simulink model "saccha"  (Simulink 6.4)
settings: Solver=ode15s  StartTime=0.0  StopTime=35  FixedStep=1  RelTol=1e-3
values from neighbouring files (symbols this model uses):
  med_err = 5    [saccha.mat]    (also in simule.m)
  r = [66 49 41 5 78 55 23 52 31 162]    [saccha.mat]    (also in simule.m = round(abs(100*randn(10,1))))
settings Model: LastModifiedBy=jcamacho
settings DataIOCC: LimitDataPoints=off  SignalLoggingName=sigsOut
settings DebuggingCC: SolverPrmCheckMsg=none  StrictBusMsg=None
settings HardwareCC: TargetUnknown=on

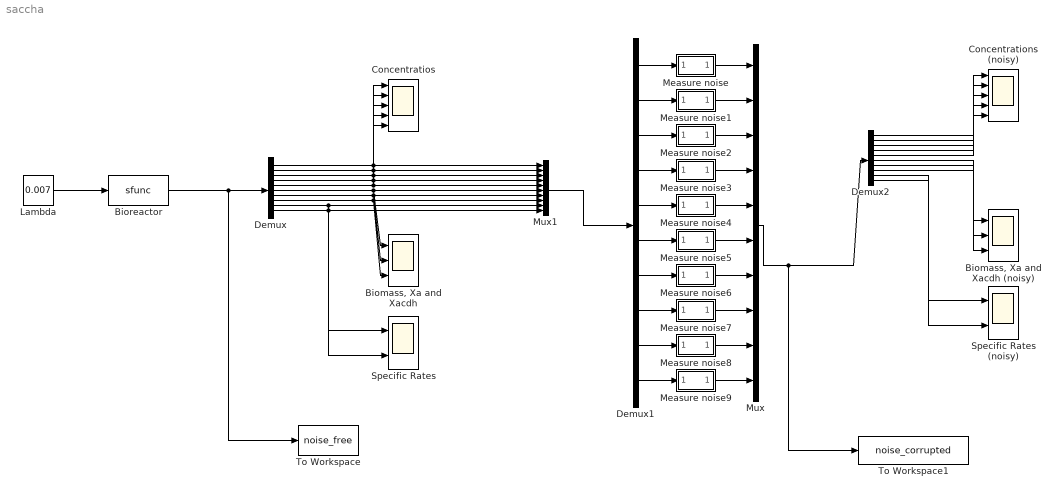
== system saccha ==
  "Biomass, Xa and Xacdh " : Scope  NumInputPorts=3
      settings: TimeRange=10  YMin=28.8275~0.9~1  YMax=28.86~1~1.04  MaxDataPoints=100000
  "Biomass, Xa and Xacdh (noisy)" : Scope  NumInputPorts=3
      settings: TimeRange=10  YMin=0.6~0.9~1  YMax=1~1~1.04  SaveName=ScopeData3  MaxDataPoints=40000
  Bioreactor : S-Function  FunctionName=sfunc  Parameters=xini, k1h, K1h, k1l, K1l, k1e, K1e, K1i, k2, K2, K2i, k3, K3, k4, K4, k5, K5, k5e, K5e, K5i, k6, K6, k6r, K6e, k7, K7, k8, k9, K9, k9e, K9e, K9i, k9c, k10, K10, k10e, K10e, k11, Sf, w, var_ini
  Concentrations (noisy) : Scope  NumInputPorts=5
      settings: TimeRange=10  YMin=0.6~0.9~1~1~0  YMax=1~1~1.04~1.001~100  SaveName=ScopeData5  MaxDataPoints=40000
  Concentratios : Scope  NumInputPorts=5
      settings: TimeRange=1  YMin=0.6~0.9~1~1~0  YMax=1~1~1.04~1.001~100  MaxDataPoints=40000
  Demux : Demux  Outputs=10
  Demux1 : Demux  Outputs=10
  Demux2 : Demux  Outputs=10
  Lambda : Constant  Value=0.007  OutDataType=sfix(16)  ConRadixGroup=Use specified scaling  OutScaling=2^0  SampleTime=inf  FramePeriod=inf
  Measure noise : Subsystem  TreatAsAtomicUnit=on  mask{v1=0, v2=15*med_err/200, v3=0, v4=r(1)}
      mask prompts: v1 "Media error blanco"; v2 "Desviacion Tipica error blanco"; v3 "Constante de error proporcional"; v4 "Semilla"
      mask init:
      | media = v1;
      | varianza = v2*v2;
      | proporcional = v3;
      | r = v4;
  Measure noise1 : Subsystem  TreatAsAtomicUnit=on  mask{v1=0, v2=0.02*med_err/200, v3=0, v4=r(2)}
      mask prompts: v1 "Media error blanco"; v2 "Desviacion Tipica error blanco"; v3 "Constante de error proporcional"; v4 "Semilla"
      mask init:
      | media = v1;
      | varianza = v2*v2;
      | proporcional = v3;
      | r = v4;
  Measure noise2 : Subsystem  TreatAsAtomicUnit=on  mask{v1=0, v2=1*med_err/200, v3=0, v4=r(3)}
      mask prompts: v1 "Media error blanco"; v2 "Desviacion Tipica error blanco"; v3 "Constante de error proporcional"; v4 "Semilla"
      mask init:
      | media = v1;
      | varianza = v2*v2;
      | proporcional = v3;
      | r = v4;
  Measure noise3 : Subsystem  TreatAsAtomicUnit=on  mask{v1=0, v2=0.05*med_err/200, v3=0, v4=r(4)}
      mask prompts: v1 "Media error blanco"; v2 "Desviacion Tipica error blanco"; v3 "Constante de error proporcional"; v4 "Semilla"
      mask init:
      | media = v1;
      | varianza = v2*v2;
      | proporcional = v3;
      | r = v4;
  Measure noise4 : Subsystem  TreatAsAtomicUnit=on  mask{v1=0, v2=5*med_err/200, v3=0, v4=r(5)}
      mask prompts: v1 "Media error blanco"; v2 "Desviacion Tipica error blanco"; v3 "Constante de error proporcional"; v4 "Semilla"
      mask init:
      | media = v1;
      | varianza = v2*v2;
      | proporcional = v3;
      | r = v4;
  Measure noise5 : Subsystem  TreatAsAtomicUnit=on  mask{v1=0, v2=2.5*med_err/200, v3=0, v4=r(6)}
      mask prompts: v1 "Media error blanco"; v2 "Desviacion Tipica error blanco"; v3 "Constante de error proporcional"; v4 "Semilla"
      mask init:
      | media = v1;
      | varianza = v2*v2;
      | proporcional = v3;
      | r = v4;
  Measure noise6 : Subsystem  TreatAsAtomicUnit=on  mask{v1=0, v2=0.1*med_err/200, v3=0, v4=r(7)}
      mask prompts: v1 "Media error blanco"; v2 "Desviacion Tipica error blanco"; v3 "Constante de error proporcional"; v4 "Semilla"
      mask init:
      | media = v1;
      | varianza = v2*v2;
      | proporcional = v3;
      | r = v4;
  Measure noise7 : Subsystem  TreatAsAtomicUnit=on  mask{v1=0, v2=0.02*med_err/200, v3=0, v4=r(8)}
      mask prompts: v1 "Media error blanco"; v2 "Desviacion Tipica error blanco"; v3 "Constante de error proporcional"; v4 "Semilla"
      mask init:
      | media = v1;
      | varianza = v2*v2;
      | proporcional = v3;
      | r = v4;
  Measure noise8 : Subsystem  TreatAsAtomicUnit=on  mask{v1=0, v2=5*med_err/200, v3=0, v4=r(9)}
      mask prompts: v1 "Media error blanco"; v2 "Desviacion Tipica error blanco"; v3 "Constante de error proporcional"; v4 "Semilla"
      mask init:
      | media = v1;
      | varianza = v2*v2;
      | proporcional = v3;
      | r = v4;
  Measure noise9 : Subsystem  TreatAsAtomicUnit=on  mask{v1=0, v2=15*med_err/200, v3=0, v4=r(10)}
      mask prompts: v1 "Media error blanco"; v2 "Desviacion Tipica error blanco"; v3 "Constante de error proporcional"; v4 "Semilla"
      mask init:
      | media = v1;
      | varianza = v2*v2;
      | proporcional = v3;
      | r = v4;
  Mux : Mux  Inputs=10
  Mux1 : Mux  Inputs=10
  Specific Rates : Scope  NumInputPorts=2
      settings: TimeRange=10  YMin=0.6~1.38778e-017  YMax=1~0.375  SaveName=ScopeData2  MaxDataPoints=40000
  Specific Rates (noisy) : Scope  NumInputPorts=2
      settings: TimeRange=10  YMin=0.6~0.9  YMax=1~1  SaveName=ScopeData4  MaxDataPoints=40000
  To Workspace : ToWorkspace  VariableName=noise_free  SampleTime=-1  SaveFormat=Structure With Time
  To Workspace1 : ToWorkspace  VariableName=noise_corrupted  SampleTime=-1  SaveFormat=Structure With Time
  wires:
  Demux/1 -> Concentratios/1, Mux1/1
  Demux/2 -> Concentratios/2, Mux1/2
  Demux/3 -> Concentratios/3, Mux1/3
  Demux/4 -> Concentratios/4, Mux1/4
  Demux/5 -> Concentratios/5, Mux1/5
  Demux/6 -> "Biomass, Xa and Xacdh "/1, Mux1/6
  Demux/7 -> "Biomass, Xa and Xacdh "/2, Mux1/7
  Demux/8 -> "Biomass, Xa and Xacdh "/3, Mux1/8
  Bioreactor/1 -> Demux/1, To Workspace/1
  Demux1/1 -> Measure noise/1(In1)
  Demux1/2 -> Measure noise1/1(In1)
  Demux1/3 -> Measure noise2/1(In1)
  Demux1/4 -> Measure noise3/1(In1)
  Demux1/5 -> Measure noise4/1(In1)
  Demux1/6 -> Measure noise5/1(In1)
  Demux1/7 -> Measure noise6/1(In1)
  Demux1/8 -> Measure noise7/1(In1)
  Measure noise/1(Out1) -> Mux/1
  Measure noise1/1(Out1) -> Mux/2
  Measure noise2/1(Out1) -> Mux/3
  Measure noise3/1(Out1) -> Mux/4
  Measure noise4/1(Out1) -> Mux/5
  Measure noise5/1(Out1) -> Mux/6
  Measure noise6/1(Out1) -> Mux/7
  Measure noise7/1(Out1) -> Mux/8
  Measure noise8/1(Out1) -> Mux/9
  Measure noise9/1(Out1) -> Mux/10
  Demux2/1 -> Concentrations (noisy)/1
  Demux2/2 -> Concentrations (noisy)/2
  Demux2/3 -> Concentrations (noisy)/3
  Demux2/4 -> Concentrations (noisy)/4
  Demux2/5 -> Concentrations (noisy)/5
  Demux2/6 -> "Biomass, Xa and Xacdh (noisy)"/1
  Demux2/7 -> "Biomass, Xa and Xacdh (noisy)"/2
  Demux2/8 -> "Biomass, Xa and Xacdh (noisy)"/3
  Demux2/9 -> Specific Rates (noisy)/1
  Demux2/10 -> Specific Rates (noisy)/2
  Mux/1 -> Demux2/1, To Workspace1/1
  Demux1/9 -> Measure noise8/1(In1)
  Demux1/10 -> Measure noise9/1(In1)
  Demux/9 -> Specific Rates/1, Mux1/9
  Demux/10 -> Specific Rates/2, Mux1/10
  Mux1/1 -> Demux1/1
  Lambda/1 -> Bioreactor/1

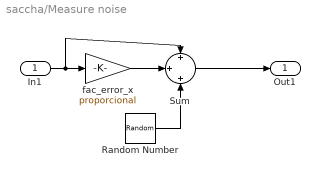
== system saccha/Measure noise ==
  In1 : Inport
  Random Number : RandomNumber  Mean=media  Variance=varianza  Seed=r  SampleTime=0
  Sum : Sum  Inputs=+|+|+  SaturateOnIntegerOverflow=on
  fac_error_x : Gain  Gain=proporcional  SaturateOnIntegerOverflow=on
  Out1 : Outport
  wires:
  Random Number/1 -> Sum/3
  In1/1 -> fac_error_x/1, Sum/1
  fac_error_x/1 -> Sum/2
  Sum/1 -> Out1/1

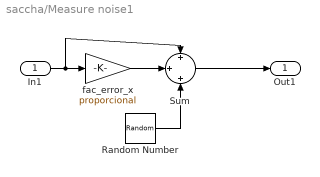
== system saccha/Measure noise1 ==
  In1 : Inport
  Random Number : RandomNumber  Mean=media  Variance=varianza  Seed=r  SampleTime=0
  Sum : Sum  Inputs=+|+|+  SaturateOnIntegerOverflow=on
  fac_error_x : Gain  Gain=proporcional  SaturateOnIntegerOverflow=on
  Out1 : Outport
  wires:
  Random Number/1 -> Sum/3
  In1/1 -> fac_error_x/1, Sum/1
  fac_error_x/1 -> Sum/2
  Sum/1 -> Out1/1

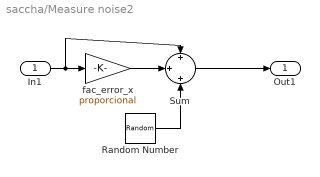
== system saccha/Measure noise2 ==
  In1 : Inport
  Random Number : RandomNumber  Mean=media  Variance=varianza  Seed=r  SampleTime=0
  Sum : Sum  Inputs=+|+|+  SaturateOnIntegerOverflow=on
  fac_error_x : Gain  Gain=proporcional  SaturateOnIntegerOverflow=on
  Out1 : Outport
  wires:
  Random Number/1 -> Sum/3
  In1/1 -> fac_error_x/1, Sum/1
  fac_error_x/1 -> Sum/2
  Sum/1 -> Out1/1

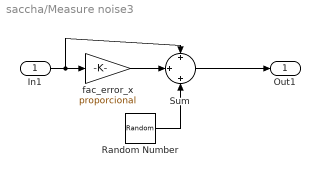
== system saccha/Measure noise3 ==
  In1 : Inport
  Random Number : RandomNumber  Mean=media  Variance=varianza  Seed=r  SampleTime=0
  Sum : Sum  Inputs=+|+|+  SaturateOnIntegerOverflow=on
  fac_error_x : Gain  Gain=proporcional  SaturateOnIntegerOverflow=on
  Out1 : Outport
  wires:
  Random Number/1 -> Sum/3
  In1/1 -> fac_error_x/1, Sum/1
  fac_error_x/1 -> Sum/2
  Sum/1 -> Out1/1

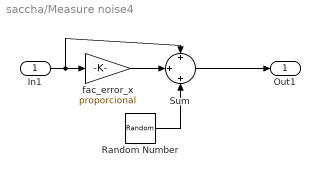
== system saccha/Measure noise4 ==
  In1 : Inport
  Random Number : RandomNumber  Mean=media  Variance=varianza  Seed=r  SampleTime=0
  Sum : Sum  Inputs=+|+|+  SaturateOnIntegerOverflow=on
  fac_error_x : Gain  Gain=proporcional  SaturateOnIntegerOverflow=on
  Out1 : Outport
  wires:
  Random Number/1 -> Sum/3
  In1/1 -> fac_error_x/1, Sum/1
  fac_error_x/1 -> Sum/2
  Sum/1 -> Out1/1

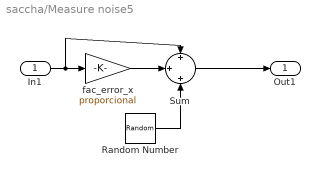
== system saccha/Measure noise5 ==
  In1 : Inport
  Random Number : RandomNumber  Mean=media  Variance=varianza  Seed=r  SampleTime=0
  Sum : Sum  Inputs=+|+|+  SaturateOnIntegerOverflow=on
  fac_error_x : Gain  Gain=proporcional  SaturateOnIntegerOverflow=on
  Out1 : Outport
  wires:
  Random Number/1 -> Sum/3
  In1/1 -> fac_error_x/1, Sum/1
  fac_error_x/1 -> Sum/2
  Sum/1 -> Out1/1

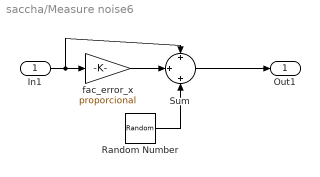
== system saccha/Measure noise6 ==
  In1 : Inport
  Random Number : RandomNumber  Mean=media  Variance=varianza  Seed=r  SampleTime=0
  Sum : Sum  Inputs=+|+|+  SaturateOnIntegerOverflow=on
  fac_error_x : Gain  Gain=proporcional  SaturateOnIntegerOverflow=on
  Out1 : Outport
  wires:
  Random Number/1 -> Sum/3
  In1/1 -> fac_error_x/1, Sum/1
  fac_error_x/1 -> Sum/2
  Sum/1 -> Out1/1

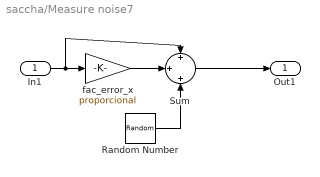
== system saccha/Measure noise7 ==
  In1 : Inport
  Random Number : RandomNumber  Mean=media  Variance=varianza  Seed=r  SampleTime=0
  Sum : Sum  Inputs=+|+|+  SaturateOnIntegerOverflow=on
  fac_error_x : Gain  Gain=proporcional  SaturateOnIntegerOverflow=on
  Out1 : Outport
  wires:
  Random Number/1 -> Sum/3
  In1/1 -> fac_error_x/1, Sum/1
  fac_error_x/1 -> Sum/2
  Sum/1 -> Out1/1

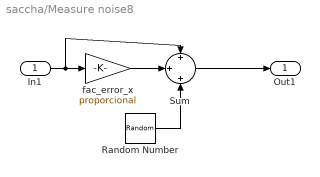
== system saccha/Measure noise8 ==
  In1 : Inport
  Random Number : RandomNumber  Mean=media  Variance=varianza  Seed=r  SampleTime=0
  Sum : Sum  Inputs=+|+|+  SaturateOnIntegerOverflow=on
  fac_error_x : Gain  Gain=proporcional  SaturateOnIntegerOverflow=on
  Out1 : Outport
  wires:
  Random Number/1 -> Sum/3
  In1/1 -> fac_error_x/1, Sum/1
  fac_error_x/1 -> Sum/2
  Sum/1 -> Out1/1

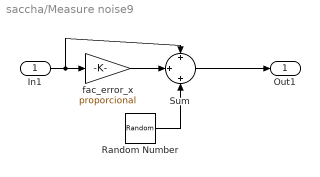
== system saccha/Measure noise9 ==
  In1 : Inport
  Random Number : RandomNumber  Mean=media  Variance=varianza  Seed=r  SampleTime=0
  Sum : Sum  Inputs=+|+|+  SaturateOnIntegerOverflow=on
  fac_error_x : Gain  Gain=proporcional  SaturateOnIntegerOverflow=on
  Out1 : Outport
  wires:
  Random Number/1 -> Sum/3
  In1/1 -> fac_error_x/1, Sum/1
  fac_error_x/1 -> Sum/2
  Sum/1 -> Out1/1
